simulink model "sistema_tema_8"  (Simulink 7.0)
settings: Solver=FixedStepDiscrete  StartTime=0.0  StopTime=10  RelTol=1e-3
undefined symbols (not defined in the file or in its folder): A, B, B0, C, H, K, T
settings Model: Creator=up  LastModifiedBy=up

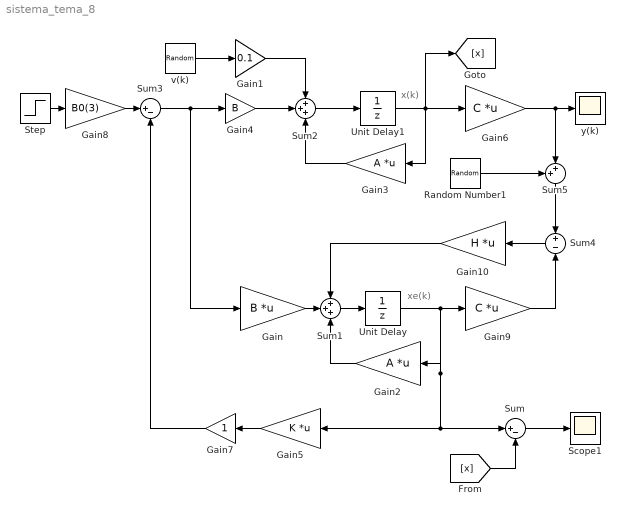
== system sistema_tema_8 ==
  note: x(k)
  note: xe(k)
  Gain : Gain  Gain=B  Multiplication=Matrix(K*u) (u vector)  ParameterDataType=sfix(16)  ParameterScaling=2^0  OutDataType=sfix(16)  OutScaling=2^0
  Gain1 : Gain  Gain=0.1  ParameterDataType=sfix(16)  ParameterScaling=2^0  OutDataType=sfix(16)  OutScaling=2^0  SampleTime=T
  Gain10 : Gain  Orientation=left  Gain=H  Multiplication=Matrix(K*u) (u vector)  ParameterDataType=sfix(16)  ParameterScaling=2^0  OutDataType=sfix(16)  OutScaling=2^0
  Gain2 : Gain  Orientation=left  Gain=A  Multiplication=Matrix(K*u) (u vector)  ParameterDataType=sfix(16)  ParameterScaling=2^0  OutDataType=sfix(16)  OutScaling=2^0
  Gain3 : Gain  Orientation=left  Gain=A  Multiplication=Matrix(K*u) (u vector)  ParameterDataType=sfix(16)  ParameterScaling=2^0  OutDataType=sfix(16)  OutScaling=2^0  SampleTime=T
  Gain4 : Gain  Gain=B  ParameterDataType=sfix(16)  ParameterScaling=2^0  OutDataType=sfix(16)  OutScaling=2^0
  Gain5 : Gain  Orientation=left  Gain=K  Multiplication=Matrix(K*u) (u vector)  ParameterDataType=sfix(16)  ParameterScaling=2^0  OutDataType=sfix(16)  OutScaling=2^0
  Gain6 : Gain  Gain=C  Multiplication=Matrix(K*u) (u vector)  ParameterDataType=sfix(16)  ParameterScaling=2^0  OutDataType=sfix(16)  OutScaling=2^0  SampleTime=T
  Gain7 : Gain  Orientation=left  ParameterDataType=sfix(16)  ParameterScaling=2^0  OutDataType=sfix(16)  OutScaling=2^0  SampleTime=T
  Gain8 : Gain  Gain=B0(3)  ParameterDataType=sfix(16)  ParameterScaling=2^0  OutDataType=sfix(16)  OutScaling=2^0
  Gain9 : Gain  Gain=C  Multiplication=Matrix(K*u) (u vector)  ParameterDataType=sfix(16)  ParameterScaling=2^0  OutDataType=sfix(16)  OutScaling=2^0
  Random Number1 : RandomNumber  Variance=0.01  SampleTime=0
  Scope1 : Scope
  Step : Step  After=10  SampleTime=0
  Sum : Sum  Inputs=|+-  OutDataType=sfix(16)  OutScaling=2^0
  Sum1 : Sum  Inputs=+++  OutDataType=sfix(16)  OutScaling=2^0
  Sum2 : Sum  Inputs=+++  OutDataType=sfix(16)  OutScaling=2^0
  Sum3 : Sum  Inputs=|+-  OutDataType=sfix(16)  OutScaling=2^0
  Sum4 : Sum  Orientation=left  Inputs=+|-  OutDataType=sfix(16)  OutScaling=2^0  SampleTime=T
  Sum5 : Sum  Orientation=down  Inputs=++|  OutDataType=sfix(16)  OutScaling=2^0
  Unit Delay : UnitDelay  X0=[0 0 0]  SampleTime=T
  Unit Delay1 : UnitDelay  X0=[randn randn randn]*10  SampleTime=T
  v(k) : RandomNumber  Mean=[0 0 0]  Variance=[1 1 1]  Seed=[0 31415 9143]  SampleTime=T
  y(k) : Scope
      settings: TimeRange=10  YMax=15  SaveName=y  DataFormat=Array
  wires:
  Gain4/1 -> Sum2/2
  Sum2/1 -> Unit Delay1/1
  Unit Delay1/1 -> Gain3/1, Gain6/1, [x]
  Gain3/1 -> Sum2/3
  v(k)/1 -> Gain1/1
  Sum3/1 -> Gain4/1, Gain/1
  Gain5/1 -> Gain7/1
  Step/1 -> Gain8/1
  Gain6/1 -> y(k)/1, Sum5/2
  Gain7/1 -> Sum3/2
  Gain8/1 -> Sum3/1
  Gain1/1 -> Sum2/1
  Sum1/1 -> Unit Delay/1
  Unit Delay/1 -> Gain9/1, Gain2/1, Gain5/1, Sum/1
  Gain9/1 -> Sum4/2
  Sum4/1 -> Gain10/1
  Gain/1 -> Sum1/2
  Gain10/1 -> Sum1/1
  Gain2/1 -> Sum1/3
  Sum/1 -> Scope1/1
  [x] -> Sum/2
  Sum5/1 -> Sum4/1
  Random Number1/1 -> Sum5/1
